simulink model "drone_5DOF_observer"  (R2023b)
settings: Solver=ode45  StartTime=0.0  StopTime=duration  MaxStep=0.001  RelTol=1e-3
values from neighbouring files (symbols this model uses):
  A = [-qr-qu,0,0,0 ... (first row only)    [partA.m]    (also in partB.m = zeros(10,10))
  B = [1,0;0,0;0,1;0,0]    [partA.m]    (also in partB.m = zeros(10,3))
  Cob = C    [partB.m]
  g = 9.81    [partB.m]
  Ki = zeros(3,7)    [partB.m]
  Kp = zeros(3,7)    [partB.m]
  L = K_duo'    [partB.m]
  mass = 0.1    [partB.m]
  x0 = zeros(10,1)    [homogeniuos.m]    (also in partB.m = randn(n,1).*[1,1,1,1,1,1,0.1,0.1,0,0]'*1; plotSimulation.m = randn(n,1)/100)
undefined symbols (not defined in the file or in its folder): K
settings Model: Creator=Shadow  LastModifiedBy=Shadow

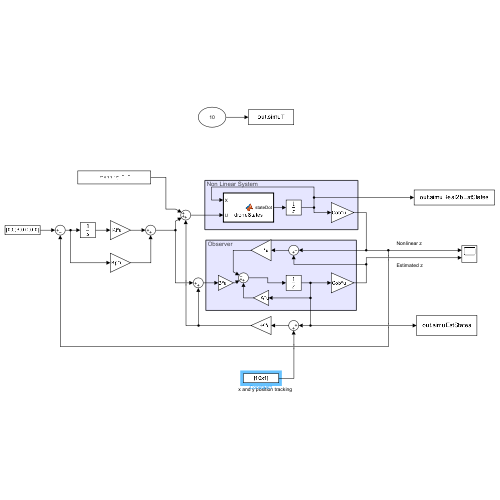
[thumbnail: Simulink's stored preview of the top-level diagram]
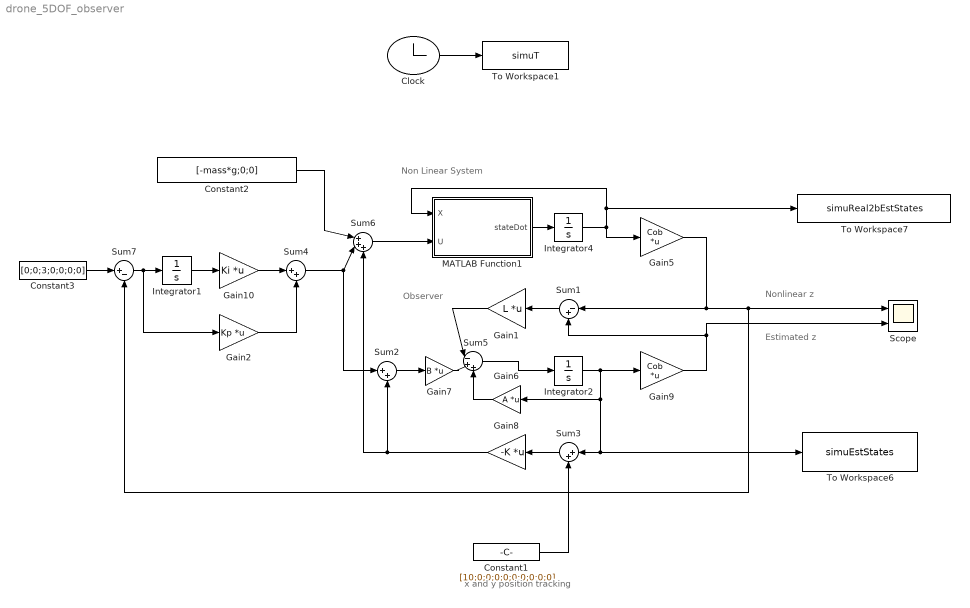
== system drone_5DOF_observer ==
  note: x and y position tracking
  note: Nonlinear z
  note: Observer
  note: Non Linear System
  note: Estimated z
  Clock : Clock
  Constant1 : Constant  Value=[10;0;0;0;0;0;0;0;0;0]
  Constant2 : Constant  Value=[-mass*g;0;0]
  Constant3 : Constant  Value=[0;0;3;0;0;0;0]
  Gain1 : Gain  Gain=L  Multiplication=Matrix(K*u)
  Gain10 : Gain  Gain=Ki  Multiplication=Matrix(K*u)
  Gain2 : Gain  Gain=Kp  Multiplication=Matrix(K*u)
  Gain5 : Gain  Gain=Cob  Multiplication=Matrix(K*u)
  Gain6 : Gain  Gain=A  Multiplication=Matrix(K*u)
  Gain7 : Gain  Gain=B  Multiplication=Matrix(K*u)
  Gain8 : Gain  Gain=-K  Multiplication=Matrix(K*u)
  Gain9 : Gain  Gain=Cob  Multiplication=Matrix(K*u)
  Integrator1 : Integrator
  Integrator2 : Integrator  InitialCondition=x0
  Integrator4 : Integrator  InitialCondition=x0
  MATLAB Function1 : MATLAB Function  TreatAsAtomicUnit=on
  Scope : Scope  NumInputPorts=2
  Sum1 : Sum  Inputs=|-+
  Sum2 : Sum  Inputs=|++
  Sum3 : Sum  Inputs=|++
  Sum4 : Sum  Inputs=|++
  Sum5 : Sum  Inputs=|-++
  Sum6 : Sum  Inputs=|+++
  Sum7 : Sum  Inputs=|+-
  To Workspace1 : ToWorkspace  VariableName=simuT  SampleTime=0.01
      settings: Save2DSignal=2-D array (concatenate along first dimension)
  To Workspace6 : ToWorkspace  VariableName=simuEstStates  SampleTime=0.01
      settings: Save2DSignal=2-D array (concatenate along first dimension)
  To Workspace7 : ToWorkspace  VariableName=simuReal2bEstStates  SampleTime=0.01
      settings: Save2DSignal=2-D array (concatenate along first dimension)
  wires:
  Gain8/1 -> Sum2/2, Sum6/3
  MATLAB Function1/1(stateDot) -> Integrator4/1
  Integrator2/1 -> Gain9/1, Sum3/1, To Workspace6/1, Gain6/1
  Sum5/1 -> Integrator2/1
  Sum6/1 -> MATLAB Function1/2(U)
  Integrator4/1 -> MATLAB Function1/1(X), To Workspace7/1, Gain5/1
  Constant2/1 -> Sum6/1
  Clock/1 -> To Workspace1/1
  Gain6/1 -> Sum5/3
  Gain7/1 -> Sum5/2
  Gain5/1 -> Sum7/2, Scope/1, Sum1/1
  Gain9/1 -> Scope/2, Sum1/2
  Sum1/1 -> Gain1/1
  Gain1/1 -> Sum5/1
  Sum2/1 -> Gain7/1
  Sum3/1 -> Gain8/1
  Constant1/1 -> Sum3/2
  Integrator1/1 -> Gain10/1
  Sum7/1 -> Gain2/1, Integrator1/1
  Constant3/1 -> Sum7/1
  Gain10/1 -> Sum4/1
  Sum4/1 -> Sum2/1, Sum6/2
  Gain2/1 -> Sum4/2

== matlab function drone_5DOF_observer/MATLAB Function1 ==
  data: X input size=10; stateDot output; U input size=3
function stateDot=droneStates(X,U)
g=9.81;
mass = 0.1;
Ix = 1e-4;
Iy = 1e-4;

x=X(1);
y=X(2);
z=X(3);
xdot=X(4);
ydot=X(5);
zdot=X(6);
phi=X(7);
theta=X(8);
phidot=X(9);
thetadot=X(10);
ft=U(1);
taux=U(2);
tauy=U(3);



stateDot=[xdot;
    ydot; 
    zdot;
    -thetadot*zdot-g*sin(theta);
    phidot*zdot+g*cos(theta)*sin(phi);
    thetadot*xdot-phidot*ydot+g*cos(theta)*cos(phi)-ft/mass;
    phidot;
    thetadot;
    taux/Ix;
    tauy/Iy];
% 
% stateDot=[xdot;
%     ydot; 
%     zdot;
%     -ft/mass*cos(phi)*sin(theta);
%     ft/mass*sin(theta);
%     g-ft/mass*(cos(phi)*cos(theta));
%     phidot;
%     thetadot;    
%     taux/Ix;
%     tauy/Iy];
